simulink library "Ampere_Library"  (R2022b)
settings: Solver=FixedStepDiscrete  StartTime=0  StopTime=10.0  RelTol=1e-3  EnableMultiTasking=on
undefined symbols (not defined in the file or in its folder): A_INST_double, Dem_EventStatusType, ECU_AMBIENT_TEMPERATURE, SET_ECU_AMBIENT_TEMPERATURE, SlDemoSign, Std_ReturnType
libraries: simulink x13
(part 10 of 10)

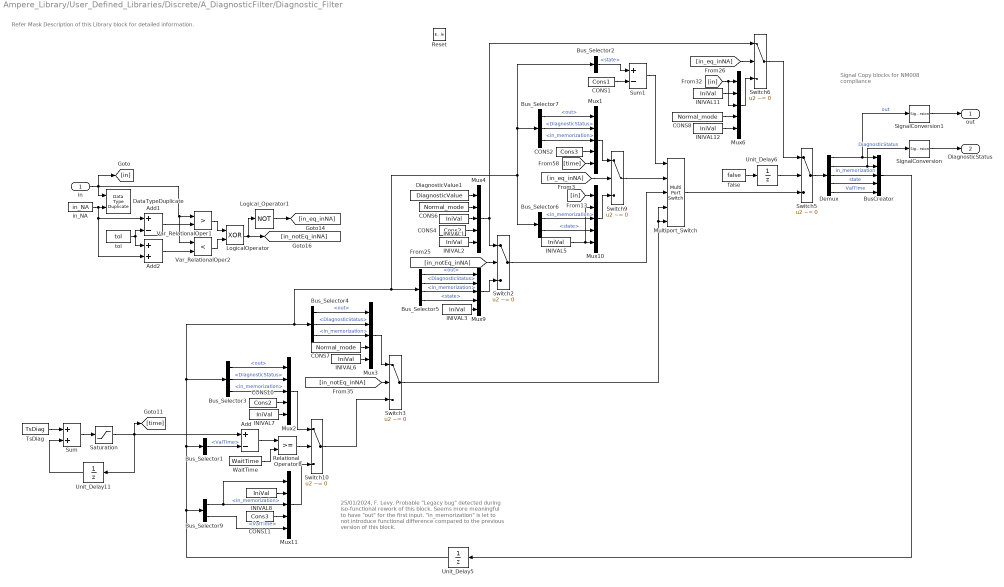
== system Ampere_Library/User_Defined_Libraries/Discrete/A_DiagnosticFilter/Diagnostic_Filter ==
  note: Signal Copy blocks for
      | NM008 compliance
  note: Refer Mask Description of this Library block for detailed information.
  note: 25/01/2024, F. Levy.
      | Probable "Legacy bug" detected
      | during iso-functional rework of this block.
      | Seems more meaningful to have "out" for the first input.
      | "in_memorization" is let to not introduce functional
      | difference compared to the previous version of this block.
  in : Inport
  Reset : EnablePort  StatesWhenEnabling=reset
      settings: AttributesFormatString=%<StatesWhenEnabling>
  Add : Sum  Inputs=+-  InputSameDT=on  RndMeth=Zero
  Add1 : Sum  Inputs=+-  InputSameDT=on  OutDataTypeStr=Inherit: Inherit via back propagation  RndMeth=Zero
  Add2 : Sum  InputSameDT=on  OutDataTypeStr=Inherit: Inherit via back propagation  RndMeth=Zero
  BusCreator : BusCreator  Inputs=5
  Bus_Selector1 : BusSelector  OutputSignals=ValTime
  Bus_Selector2 : BusSelector  OutputSignals=state
  Bus_Selector3 : BusSelector  OutputSignals=out,DiagnosticStatus,in_memorization
  Bus_Selector4 : BusSelector  OutputSignals=out,DiagnosticStatus,in_memorization
  Bus_Selector5 : BusSelector  OutputSignals=out,DiagnosticStatus,in_memorization,state
  Bus_Selector6 : BusSelector  OutputSignals=in_memorization,state
  Bus_Selector7 : BusSelector  OutputSignals=out,DiagnosticStatus,in_memorization
  Bus_Selector9 : BusSelector  OutputSignals=in_memorization,ValTime
  CONS1 : Constant  Value=Cons1  OutDataTypeStr=Inherit: Inherit via back propagation
  CONS10 : Constant  Value=Cons2  OutDataTypeStr=Inherit: Inherit via back propagation
  CONS11 : Constant  Value=Cons3  OutDataTypeStr=Inherit: Inherit via back propagation
  CONS2 : Constant  Value=Cons3  OutDataTypeStr=Inherit: Inherit via back propagation
  CONS4 : Constant  Value=Cons2  OutDataTypeStr=Inherit: Inherit via back propagation
  CONS6 : Constant  Value=Normal_mode  OutDataTypeStr=Inherit: Inherit via back propagation
  CONS7 : Constant  Value=Normal_mode  OutDataTypeStr=Inherit: Inherit via back propagation
  CONS8 : Constant  Value=Normal_mode  OutDataTypeStr=Inherit: Inherit via back propagation
  DataTypeDuplicate : DataTypeDuplicate
  Demux : Demux  Outputs=5
  DiagnosticValue1 : Constant  Value=DiagnosticValue  OutDataTypeStr=Inherit: Inherit via back propagation
  INIVAL{1..3,5..8,11..12} (9 alike) : Constant  Value=IniVal  OutDataTypeStr=Inherit: Inherit via back propagation
  LogicalOperator : Logic  Operator=XOR  OutDataTypeStr=boolean
  Logical_Operator1 : Logic  Operator=NOT  OutDataTypeStr=boolean
  Multiport_Switch : MultiPortSwitch  DataPortOrder=Zero-based contiguous  DataPortForDefault=Additional data port  DiagnosticForDefault=None  zeroidx=on  RndMeth=Zero  SaturateOnIntegerOverflow=off
  Mux{1..4,6,9..11} (8 alike) : Mux  Inputs=5
  Relational_Operator8 : RelationalOperator  OutDataTypeStr=boolean  RndMeth=Zero
  Saturation : Saturate  UpperLimit=UpperLimit  LowerLimit=LowerLimit  RndMeth=Zero
      settings: AttributesFormatString="Max =  %<UpperLimit>\\n Min = %<LowerLimit> \\n"
  SignalConversion : SignalConversion  OverrideOpt=off
  SignalConversion1 : SignalConversion  OverrideOpt=off
  Sum : Sum  InputSameDT=on  RndMeth=Zero
  Sum1 : Sum  Inputs=+-  InputSameDT=on  OutDataTypeStr=uint8  RndMeth=Zero  SaturateOnIntegerOverflow=on
      settings: AttributesFormatString=SAT = %<SaturateOnIntegerOverflow>\n DT = %<OutDataTypeStr>\n
  Switch{2..3,5..6,9..10} (6 alike) : Switch  Criteria=u2 ~= 0  RndMeth=Zero  SaturateOnIntegerOverflow=off
  TsDiag : Constant  Value=TsDiag  OutDataTypeStr=Inherit: Inherit via back propagation
  Unit_Delay11 : UnitDelay  InitialCondition=TsDiag_init  SampleTime=-1  HasFrameUpgradeWarning=on
      settings: AttributesFormatString=Init = %<InitialCondition>
  Unit_Delay5 : UnitDelay  InitialCondition=IniVal  SampleTime=-1  HasFrameUpgradeWarning=on
      settings: AttributesFormatString=Init = %<InitialCondition>
  Unit_Delay6 : UnitDelay  InitialCondition=true  SampleTime=-1  HasFrameUpgradeWarning=on
      settings: AttributesFormatString=Init = %<InitialCondition>
  Var_RelationalOper1 : RelationalOperator  Operator=>  OutDataTypeStr=boolean  RndMeth=Zero
  Var_RelationalOper2 : RelationalOperator  Operator=<  OutDataTypeStr=boolean  RndMeth=Zero
  WaitTime : Constant  Value=WaitTime  OutDataTypeStr=Inherit: Inherit via back propagation
  false : Constant  Value=false
  in_NA : Constant  Value=in_NA  OutDataTypeStr=Inherit: Inherit via back propagation
  tol : Constant  Value=tol  OutDataTypeStr=Inherit: Inherit via back propagation
  out : Outport  OutputWhenDisabled=reset  InitialOutput=DefaultValue
      settings: AttributesFormatString=Init = %<InitialOutput>\n %<OutputWhenDisabled>\n
  DiagnosticStatus : Outport  Port=2  OutputWhenDisabled=reset  InitialOutput=IniVal
      settings: AttributesFormatString=Init = %<InitialOutput>\n %<OutputWhenDisabled>\n
  wires:
  Bus_Selector9/2 -> Mux11/5  "<ValTime>"
  SignalConversion1/1 -> out/1
  SignalConversion/1 -> DiagnosticStatus/1
  Bus_Selector7/3 -> Mux1/3  "<in_memorization>"
  Bus_Selector7/2 -> Mux1/2  "<DiagnosticStatus>"
  Bus_Selector7/1 -> Mux1/1  "<out>"
  Bus_Selector6/2 -> Mux10/4  "<state>"
  Bus_Selector6/1 -> Mux10/3  "<in_memorization>"
  Bus_Selector5/4 -> Mux9/4  "<state>"
  Bus_Selector5/3 -> Mux9/3  "<in_memorization>"
  Bus_Selector5/2 -> Mux9/2  "<DiagnosticStatus>"
  Bus_Selector5/1 -> Mux9/1  "<out>"
  Bus_Selector4/3 -> Mux3/3  "<in_memorization>"
  Bus_Selector4/2 -> Mux3/2  "<DiagnosticStatus>"
  Bus_Selector4/1 -> Mux3/1  "<out>"
  Bus_Selector3/3 -> Mux2/3  "<in_memorization>"
  Bus_Selector3/1 -> Mux2/1  "<out>"
  Bus_Selector1/1 -> Add/2  "<ValTime>"
  Unit_Delay5/1 -> Bus_Selector9/1, Bus_Selector1/1, Bus_Selector3/1, Bus_Selector4/1, Bus_Selector6/1, Bus_Selector7/1, Bus_Selector2/1, Bus_Selector5/1
  BusCreator/1 -> Unit_Delay5/1
  in_NA/1 -> Add2/2, Add1/1, DataTypeDuplicate/2
  WaitTime/1 -> Relational_Operator8/2
  Demux/1 -> SignalConversion1/1, BusCreator/1  "out"
  Demux/2 -> BusCreator/2, SignalConversion/1  "DiagnosticStatus"
  INIVAL1/1 -> Mux4/3
  [in] -> Mux10/1
  Mux11/1 -> Switch10/3
  Add/1 -> Relational_Operator8/1
  Mux6/1 -> Switch6/3
  Relational_Operator8/1 -> Switch10/2
  Mux2/1 -> Switch10/1
  CONS10/1 -> Mux2/4
  Unit_Delay11/1 -> Sum/2
  Switch2/1 -> Multiport_Switch/3
  CONS8/1 -> Mux6/4
  Switch6/1 -> Switch5/1
  Add1/1 -> Var_RelationalOper1/2
  Sum1/1 -> Multiport_Switch/1
  Switch3/1 -> Multiport_Switch/5, Multiport_Switch/4
  INIVAL8/1 -> Mux11/2
  Switch9/1 -> Multiport_Switch/2
  Mux4/1 -> Switch6/1, Switch2/1
  Multiport_Switch/1 -> Switch5/3
  Mux9/1 -> Switch2/3
  LogicalOperator/1 -> [in_notEq_inNA], Logical_Operator1/1
  INIVAL3/1 -> Mux9/5
  [in] -> Mux6/1, Mux6/3
  Demux/4 -> BusCreator/4  "state"
  CONS2/1 -> Mux1/4
  Demux/3 -> BusCreator/3  "in_memorization"
  [in_notEq_inNA] -> Switch2/2
  INIVAL11/1 -> Mux6/2
  [in_eq_inNA] -> Switch9/2
  Unit_Delay6/1 -> Switch5/2
  Mux10/1 -> Switch9/3
  INIVAL5/1 -> Mux10/5, Mux10/2
  CONS7/1 -> Mux3/4
  CONS4/1 -> Mux4/4
  CONS6/1 -> Mux4/2
  Saturation/1 -> [time], Add/1, Unit_Delay11/1
  INIVAL2/1 -> Mux4/5
  Switch10/1 -> Switch3/3
  Demux/5 -> BusCreator/5  "ValTime"
  INIVAL12/1 -> Mux6/5
  Mux1/1 -> Switch9/1
  [in_notEq_inNA] -> Switch3/2
  Mux3/1 -> Switch3/1
  false/1 -> Unit_Delay6/1
  INIVAL7/1 -> Mux2/5
  Logical_Operator1/1 -> [in_eq_inNA]
  Var_RelationalOper2/1 -> LogicalOperator/2
  Bus_Selector2/1 -> Sum1/1  "<state>"
  Switch5/1 -> Demux/1
  [time] -> Mux1/5
  Add2/1 -> Var_RelationalOper2/2
  INIVAL6/1 -> Mux3/5
  tol/1 -> Add1/2, Add2/1
  CONS11/1 -> Mux11/4
  in/1 -> [in], Var_RelationalOper1/1, Var_RelationalOper2/1, DataTypeDuplicate/1
  TsDiag/1 -> Sum/1
  CONS1/1 -> Sum1/2
  Sum/1 -> Saturation/1
  Var_RelationalOper1/1 -> LogicalOperator/1
  [in_eq_inNA] -> Switch6/2
  DiagnosticValue1/1 -> Mux4/1
  Bus_Selector3/2 -> Mux2/2  "<DiagnosticStatus>"
  Bus_Selector9/1 -> Mux11/3, Mux11/1  "<in_memorization>"

== system Ampere_Library/User_Defined_Libraries/Logic_and_Bit_Operations/A_DetectChange/Float_CompInit ==
  note: abs(U-U/z)>tol
  note: Comparison for float signals
  U : Inport
  Abs : Abs  RndMeth=Zero  SaturateOnIntegerOverflow=off
  Add : Sum  Inputs=+-  InputSameDT=on  RndMeth=Zero
  Constant : Constant  Value=tol  OutDataTypeStr=Inherit: Inherit via back propagation
  Relational_Operator : RelationalOperator  Operator=>  OutDataTypeStr=boolean  RndMeth=Zero
  Unit_Delay : UnitDelay  InitialCondition=vinit  SampleTime=-1  HasFrameUpgradeWarning=on
      settings: AttributesFormatString=Init = %<InitialCondition>
  Y : Outport
  wires:
  U/1 -> Unit_Delay/1, Add/1
  Unit_Delay/1 -> Add/2
  Relational_Operator/1 -> Y/1
  Add/1 -> Abs/1
  Abs/1 -> Relational_Operator/1
  Constant/1 -> Relational_Operator/2

== system Ampere_Library/User_Defined_Libraries/Logic_and_Bit_Operations/A_DetectChange/Float_NoComp ==
  note: Outputs false at the first execution
  note: abs(U-U/z)>tol
  note: Comparison for float signals
  U : Inport
  Abs : Abs  RndMeth=Zero  SaturateOnIntegerOverflow=off
  Add : Sum  Inputs=+-  InputSameDT=on  RndMeth=Zero
  Constant : Constant  Value=tol  OutDataTypeStr=Inherit: Inherit via back propagation
  Constant1 : Constant  Value=true
  Constant2 : Constant  Value=false
  Delay_Input2 : UnitDelay  Description=Store in Global RAM  DisableCoverage=on  InitialCondition=false  SampleTime=-1  HasFrameUpgradeWarning=on
      settings: AttributesFormatString=Init = %<InitialCondition>\n
  Relational_Operator : RelationalOperator  Operator=>  OutDataTypeStr=boolean  RndMeth=Zero
  Switch : Switch  Criteria=u2 ~= 0  RndMeth=Zero  SaturateOnIntegerOverflow=off
  Unit_Delay : UnitDelay  InitialCondition=vinit  SampleTime=-1  HasFrameUpgradeWarning=on
      settings: AttributesFormatString=Init = %<InitialCondition>
  Y : Outport
  wires:
  U/1 -> Unit_Delay/1, Add/1
  Unit_Delay/1 -> Add/2
  Switch/1 -> Y/1
  Constant1/1 -> Delay_Input2/1
  Relational_Operator/1 -> Switch/1
  Constant2/1 -> Switch/3
  Delay_Input2/1 -> Switch/2
  Add/1 -> Abs/1
  Abs/1 -> Relational_Operator/1
  Constant/1 -> Relational_Operator/2

== system Ampere_Library/User_Defined_Libraries/Logic_and_Bit_Operations/A_DetectChange/NonFloat_CompInit ==
  note: Comparison for non-float signals
  U : Inport
  Relational_Operator : RelationalOperator  Operator=~=  OutDataTypeStr=boolean  RndMeth=Zero
  Unit_Delay : UnitDelay  InitialCondition=vinit  SampleTime=-1  HasFrameUpgradeWarning=on
      settings: AttributesFormatString=Init = %<InitialCondition>
  Y : Outport
  wires:
  Relational_Operator/1 -> Y/1
  Unit_Delay/1 -> Relational_Operator/2
  U/1 -> Unit_Delay/1, Relational_Operator/1

== system Ampere_Library/User_Defined_Libraries/Logic_and_Bit_Operations/A_DetectChange/NonFloat_NoComp ==
  note: Outputs false at the first execution
  note: Comparison for non-float signals
  U : Inport
  Constant1 : Constant  Value=true
  Constant2 : Constant  Value=false
  Delay_Input2 : UnitDelay  Description=Store in Global RAM  DisableCoverage=on  InitialCondition=false  SampleTime=-1  HasFrameUpgradeWarning=on
      settings: AttributesFormatString=Init = %<InitialCondition>\n
  Relational_Operator : RelationalOperator  Operator=~=  OutDataTypeStr=boolean  RndMeth=Zero
  Switch : Switch  Criteria=u2 ~= 0  RndMeth=Zero  SaturateOnIntegerOverflow=off
  Unit_Delay : UnitDelay  InitialCondition=vinit  SampleTime=-1  HasFrameUpgradeWarning=on
      settings: AttributesFormatString=Init = %<InitialCondition>
  Y : Outport
  wires:
  U/1 -> Unit_Delay/1, Relational_Operator/1
  Unit_Delay/1 -> Relational_Operator/2
  Switch/1 -> Y/1
  Constant1/1 -> Delay_Input2/1
  Relational_Operator/1 -> Switch/1
  Constant2/1 -> Switch/3
  Delay_Input2/1 -> Switch/2

== system Ampere_Library/User_Defined_Libraries/Math_Operations/A_SquareRoot/While_Iterator ==
  note: Refer Mask Description of this Library block for detailed information.
  note: A_DivisionByZero
  In : Inport
  Abs1 : Abs  RndMeth=Zero  SaturateOnIntegerOverflow=off
  Add : Sum  InputSameDT=on  RndMeth=Zero
      settings: AttributesFormatString=SAT = %<SaturateOnIntegerOverflow>
  CONS2 : Constant  Value=Cons2  OutDataTypeStr=Inherit: Inherit via back propagation
  Divide : Product  Inputs=*/  InputSameDT=on  RndMeth=Zero  SaturateOnIntegerOverflow=on
      settings: AttributesFormatString=SAT = %<SaturateOnIntegerOverflow>
  Divide1 : Product  Inputs=*/  RndMeth=Zero
  RelationalOperator : RelationalOperator  Operator=>  OutDataTypeStr=boolean  RndMeth=Zero
  RelationalOperator1 : RelationalOperator  Operator=>  OutDataTypeStr=boolean  RndMeth=Zero
  Switch : Switch  Criteria=u2 ~= 0  RndMeth=Zero  SaturateOnIntegerOverflow=off
  Switch2 : Switch  Criteria=u2 ~= 0  RndMeth=Zero  SaturateOnIntegerOverflow=off
  Unit_Delay : UnitDelay  InitialCondition=UdicVal  SampleTime=-1  HasFrameUpgradeWarning=on
      settings: AttributesFormatString=Init = %<InitialCondition>
  Unit_Delay1 : UnitDelay  InitialCondition=true  SampleTime=-1  HasFrameUpgradeWarning=on
      settings: AttributesFormatString=Init = %<InitialCondition>
  Unit_Delay3 : UnitDelay  InitialCondition=true  SampleTime=-1  HasFrameUpgradeWarning=on
      settings: AttributesFormatString=Init = %<InitialCondition>
  While_Iterator : WhileIterator  MaxIters=numofiter  WhileBlockType=do-while  ResetStates=reset  OutputDataType=int16
      settings: AttributesFormatString=Max iteration = %<MaxIters>\n %<ResetStates>\n
  cmpTol : Constant  Value=cmpTol  OutDataTypeStr=Inherit: Inherit via back propagation
  constZero : Constant  DisableCoverage=on  Value=constZero  OutDataTypeStr=Inherit: Inherit via back propagation  PreserveConstantTs=on
  false : Constant  DisableCoverage=on  Value=false  PreserveConstantTs=on
  true : Constant  DisableCoverage=on  Value=true  PreserveConstantTs=on
  Out : Outport  InitialOutput=UdicVal
      settings: AttributesFormatString=Init = %<InitialOutput>\n
  wires:
  Abs1/1 -> RelationalOperator1/1
  Unit_Delay/1 -> Add/2, Abs1/1, RelationalOperator/1, Divide1/2  "Out_z1"
  constZero/1 -> Switch/3
  cmpTol/1 -> RelationalOperator1/2
  Divide1/1 -> Switch/1
  RelationalOperator1/1 -> Switch/2
  In/1 -> Divide1/1
  Unit_Delay3/1 -> While_Iterator/1
  Divide/1 -> Unit_Delay/1, RelationalOperator/2, Out/1  "Out"
  Switch2/1 -> Unit_Delay3/1
  true/1 -> Switch2/1
  Unit_Delay1/1 -> Switch2/2
  false/1 -> Unit_Delay1/1
  RelationalOperator/1 -> Switch2/3
  Switch/1 -> Add/1
  Add/1 -> Divide/1
  CONS2/1 -> Divide/2

== system Ampere_Library/User_Defined_Libraries/Signal_Routing/A_SlopeSwitch2Inputs/Slope_On_Block ==
  note: Output_Comparision
  note: Error_Due_To_High_Slope_Test
  note: Refer Mask Description of this Library block for detailed information.
  Signal_Change : Inport
  Pos_Slope : Inport  Port=2
  Neg_Slope : Inport  Port=3
  Inp : Inport  Port=4
  Prev_Output : Inport  Port=5
  Enable_Slope_On_Block : EnablePort  StatesWhenEnabling=reset
      settings: AttributesFormatString=%<StatesWhenEnabling>\n
  Logical_Operator : Logic  Operator=OR  OutDataTypeStr=boolean
  Logical_Operator1 : Logic  Operator=OR  OutDataTypeStr=boolean
  Logical_Operator2 : Logic  OutDataTypeStr=boolean
  Product : Product  InputSameDT=on  OutDataTypeStr=Inherit: Inherit via back propagation  RndMeth=Zero
      settings: AttributesFormatString=SAT = %<SaturateOnIntegerOverflow>
  Product1 : Product  InputSameDT=on  OutDataTypeStr=Inherit: Inherit via back propagation  RndMeth=Zero
      settings: AttributesFormatString=SAT = %<SaturateOnIntegerOverflow>
  Relational_Operator1 : RelationalOperator  Operator=>  OutDataTypeStr=boolean  RndMeth=Zero
  Relational_Operator2 : RelationalOperator  Operator=<  OutDataTypeStr=boolean  RndMeth=Zero
  Relational_Operator3 : RelationalOperator  Operator=~=  OutDataTypeStr=boolean  RndMeth=Zero
  Sum : Sum  InputSameDT=on  RndMeth=Zero
  Sum1 : Sum  InputSameDT=on  RndMeth=Zero
  Switch1 : Switch  Criteria=u2 ~= 0  RndMeth=Zero  SaturateOnIntegerOverflow=off
  Switch2 : Switch  Criteria=u2 ~= 0  RndMeth=Zero  SaturateOnIntegerOverflow=off
  Switch3 : Switch  Criteria=u2 ~= 0  RndMeth=Zero  SaturateOnIntegerOverflow=off
  Unit_Delay1 : UnitDelay  InitialCondition=InitDelay  SampleTime=-1  HasFrameUpgradeWarning=on
      settings: AttributesFormatString=Init = %<InitialCondition>\n
  st : Constant  Value=st  OutDataTypeStr=Inherit: Inherit via back propagation
  Output_Not_Equals_Input : Outport  InitialOutput=false
      settings: AttributesFormatString=|
      | Init = %<InitialOutput>
      | %<OutputWhenDisabled>
  Outp : Outport  Port=2  InitialOutput=InitOut
      settings: AttributesFormatString=|
      | Init = %<InitialOutput>
      | %<OutputWhenDisabled>
  wires:
  Switch3/1 -> Outp/1  "Outp"
  Logical_Operator2/1 -> Output_Not_Equals_Input/1  "Output_Not_Equals_Input"
  Unit_Delay1/1 -> Relational_Operator3/2
  Relational_Operator3/1 -> Logical_Operator1/2
  [RelOp1_out] -> Relational_Operator3/1
  Relational_Operator2/1 -> Logical_Operator/1, Switch2/2, Unit_Delay1/1
  Signal_Change/1 -> Logical_Operator1/1
  Sum1/1 -> Switch2/1, Relational_Operator2/1
  Relational_Operator1/1 -> [RelOp1_out], Switch1/2
  Logical_Operator1/1 -> Switch3/2, Logical_Operator2/1
  Logical_Operator/1 -> Logical_Operator2/2
  Prev_Output/1 -> Sum/1, Sum1/2
  Switch1/1 -> Switch2/3
  Switch2/1 -> Switch3/1
  Inp/1 -> [Inp], Switch1/3, Relational_Operator1/2
  [Inp] -> Switch3/3
  Sum/1 -> Switch1/1, Relational_Operator1/1
  [RelOp1_out] -> Logical_Operator/2
  [Inp] -> Relational_Operator2/2
  st/1 -> Product/2, Product1/1
  Pos_Slope/1 -> Product/1
  Product/1 -> Sum1/1
  Product1/1 -> Sum/2
  Neg_Slope/1 -> Product1/2

== system Ampere_Library/User_Defined_Libraries/Timers_and_Counters/A_TurnOnDly_Ext_TimeSt/Elab_TimeStepSup ==
  note: DataType updated
      | through mask callback
  note: Evaluate the timestep
  Signal : Inport
  Timestep : Inport  Port=2
  Delaytime : Inport  Port=3
  BOOSTING_FLP : Constant  Value=Boosting_FLP  OutDataTypeStr=single
      settings: AttributesFormatString=DT = %<OutDataTypeStr>\n
  DataTypeDuplicate : DataTypeDuplicate  NumInputPorts=3
  DelayInput2 : UnitDelay  Description=\nStore in Global RAM  InitialCondition=Tim1Ini  SampleTime=-1  HasFrameUpgradeWarning=on
      settings: AttributesFormatString=Init = %<InitialCondition>\n
  DelayInput3 : UnitDelay  Description=\nStore in Global RAM  InitialCondition=initinit  SampleTime=-1  HasFrameUpgradeWarning=on
      settings: AttributesFormatString=Init = %<InitialCondition>\n
  LogicalOperator2 : Logic  OutDataTypeStr=boolean
  LogicalOperator3 : Logic  Operator=NOT  Inputs=1  OutDataTypeStr=boolean
  Product : Product  OutDataTypeStr=Inherit: Inherit via back propagation  RndMeth=Zero
      settings: AttributesFormatString=SAT = %<SaturateOnIntegerOverflow>
  Product1 : Product  OutDataTypeStr=Inherit: Inherit via back propagation  RndMeth=Zero
      settings: AttributesFormatString=SAT = %<SaturateOnIntegerOverflow>
  RelationalOperator1 : RelationalOperator  Operator=>  OutDataTypeStr=boolean  ZeroCross=off  RndMeth=Zero
  RelationalOperator2 : RelationalOperator  Operator=<=  OutDataTypeStr=boolean  ZeroCross=off  RndMeth=Zero
  Sum : Sum  Inputs=+-  InputSameDT=on  RndMeth=Zero
      settings: AttributesFormatString=SAT = %<SaturateOnIntegerOverflow>
  Switch : Switch  Criteria=u2 ~= 0  RndMeth=Zero  SaturateOnIntegerOverflow=off
  Switch2 : Switch  Criteria=u2 ~= 0  RndMeth=Zero  SaturateOnIntegerOverflow=off
  Switch4 : Switch  Criteria=u2 ~= 0  RndMeth=Zero  SaturateOnIntegerOverflow=off
  TIM1INI : Constant  Value=Tim1Ini  OutDataTypeStr=Inherit: Inherit via back propagation
  EdgeRising : Outport
  TimeStepSup : Outport  Port=2
  wires:
  [Tim1Ini] -> Switch/1
  TIM1INI/1 -> DataTypeDuplicate/3, [Tim1Ini]
  [Timestep1] -> RelationalOperator2/1, Sum/2
  Product/1 -> RelationalOperator1/1, [Timestep1]
  RelationalOperator2/1 -> Switch4/2
  Switch/1 -> DelayInput2/1
  Switch2/1 -> RelationalOperator1/2, Switch/3
  Switch4/1 -> Switch2/3
  [Tim1Ini] -> Switch4/3
  BOOSTING_FLP/1 -> Product1/1, Product/2
  Product1/1 -> Switch2/1
  Delaytime/1 -> DataTypeDuplicate/2, Product1/2
  DelayInput2/1 -> RelationalOperator2/2, Sum/1
  Sum/1 -> Switch4/1
  RelationalOperator1/1 -> Switch/2, TimeStepSup/1  "TimeStepSup"
  Timestep/1 -> DataTypeDuplicate/1, Product/1
  LogicalOperator2/1 -> Switch2/2, EdgeRising/1  "EdgeRising"
  LogicalOperator3/1 -> LogicalOperator2/2
  Signal/1 -> LogicalOperator2/1, DelayInput3/1
  DelayInput3/1 -> LogicalOperator3/1

== system Ampere_Library/User_Defined_Libraries/Timers_and_Counters/A_TurnOnDly_Ext_TimeSt/VariantInitOutput ==
  note: This variant subsystem is meant to avoid Dead Logic with the former unique implementation for the Output Init value.
  Signal : Inport
  EdgeRising : Inport  Port=2
  TimeStepSup : Inport  Port=3
  Init_false : Subsystem  VariantControl=(default)
  Init_true : Subsystem  VariantControl=Variant1
  Out : Outport

== system Ampere_Library/User_Defined_Libraries/Timers_and_Counters/A_TurnOnDly_Ext_TimeSt/VariantInitOutput/Init_false ==
  note: Case False : The init value of the unit delay is hard coded to false (= TimeOutInit set to 0)
  Signal : Inport
  EdgeRising : Inport  Port=2
  TimeStepSup : Inport  Port=3
  DelayInput1 : UnitDelay  Description=\nStore in Global RAM  InitialCondition=false  SampleTime=-1  HasFrameUpgradeWarning=on
      settings: AttributesFormatString=Init = %<InitialCondition>\n
  LogicalOperator : Logic  Inputs=3  OutDataTypeStr=boolean
  Switch1 : Switch  Criteria=u2 ~= 0  RndMeth=Zero  SaturateOnIntegerOverflow=off
  Out : Outport
  wires:
  DelayInput1/1 -> Switch1/3
  TimeStepSup/1 -> LogicalOperator/3
  Switch1/1 -> LogicalOperator/2, DelayInput1/1
  EdgeRising/1 -> Switch1/1, Switch1/2
  LogicalOperator/1 -> Out/1
  Signal/1 -> LogicalOperator/1

== system Ampere_Library/User_Defined_Libraries/Timers_and_Counters/A_TurnOnDly_Ext_TimeSt/VariantInitOutput/Init_true ==
  note: Case True : EdgeRising is not used.
  Signal : Inport
  EdgeRising : Inport  Port=2
  TimeStepSup : Inport  Port=3
  LogicalOperator : Logic  OutDataTypeStr=boolean
  Terminator : Terminator
  Out : Outport
  wires:
  EdgeRising/1 -> Terminator/1
  Signal/1 -> LogicalOperator/1
  LogicalOperator/1 -> Out/1
  TimeStepSup/1 -> LogicalOperator/2

== matlab function Ampere_Library/MBD_Base_Blocks/Simulink/User_Defined_Functions/MATLAB_Function ==
  data: u input double size=1; y output double size=1
function y = fcn(u)
% Description: Refer to MFxxx rules
y = u;

== stateflow chart Ampere_Library/MBD_Base_Blocks/Stateflow/Chart ==
  note: Default chart configured with
      | SF034 and LK012 rules compliance
  (default) -> (junction 1)
